simulink model "TRT_sim2021a"  (R2021a)
settings: Solver=VariableStepAuto  StartTime=0.0  StopTime=10.0  RelTol=1e-3
values from neighbouring files (symbols this model uses):
  g = 9.81    [RTR.m]    (also in TRT.m)
  l2 = 0.3    [RTR.m]    (also in TRT.m)
  l3 = 0.2    [RTR.m]    (also in TRT.m)
  m2 = 20    [RTR.m]    (also in TRT.m)
  m3 = 20    [RTR.m]    (also in TRT.m)
settings Model: Creator=kacpe  LastModifiedBy=kacpe
settings DebuggingCC: UnconnectedInputMsg=none  UnconnectedOutputMsg=none  UnconnectedLineMsg=none
settings RTWCC: DLArmComputeVersion=20.02.1

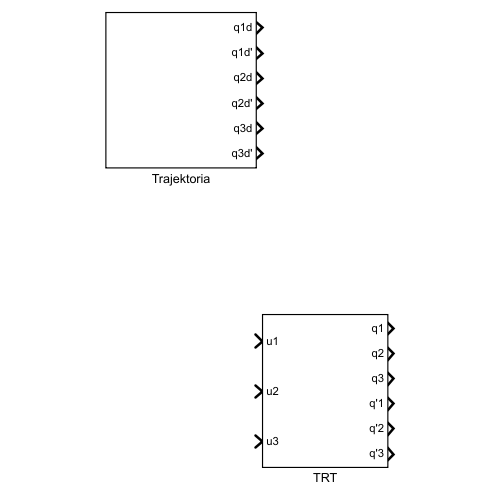
[thumbnail: Simulink's stored preview of the top-level diagram]
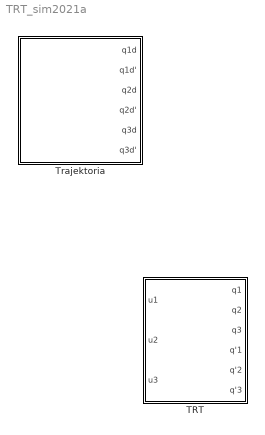
== system TRT_sim2021a ==
  TRT : Subsystem
  Trajektoria : Subsystem

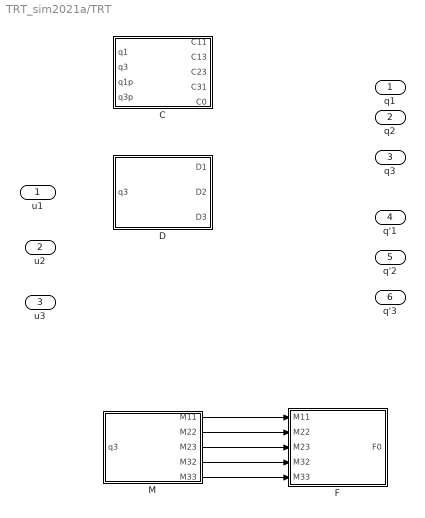
== system TRT_sim2021a/TRT ==
  u1 : Inport
  u2 : Inport  Port=2
  u3 : Inport  Port=3
  C : MATLAB Function  TreatAsAtomicUnit=on
  D : MATLAB Function  TreatAsAtomicUnit=on
  F : MATLAB Function  TreatAsAtomicUnit=on
  M : MATLAB Function  TreatAsAtomicUnit=on
  q1 : Outport
  q2 : Outport  Port=2
  q3 : Outport  Port=3
  q'1 : Outport  Port=4
  q'2 : Outport  Port=5
  q'3 : Outport  Port=6
  wires:
  M/1(M11) -> F/1(M11)
  M/2(M22) -> F/2(M22)
  M/3(M23) -> F/3(M23)
  M/4(M32) -> F/4(M32)
  M/5(M33) -> F/5(M33)

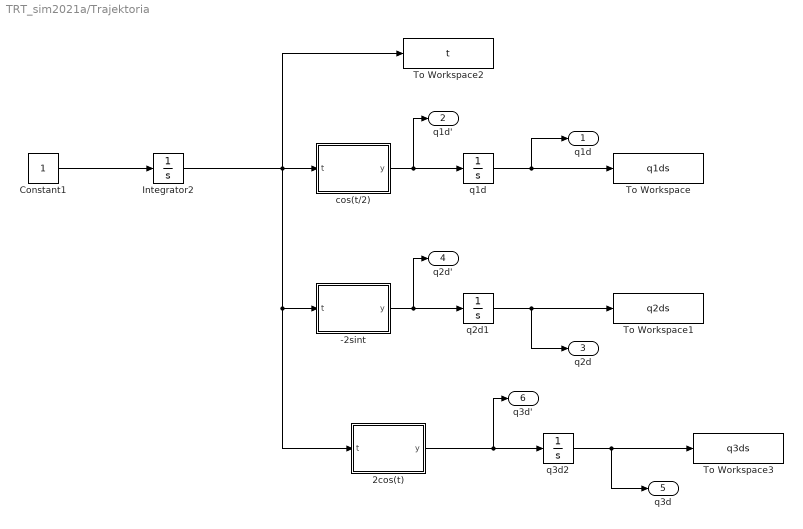
== system TRT_sim2021a/Trajektoria ==
  " q1d" : Integrator
  " q2d1" : Integrator  InitialCondition=2
  " q3d2" : Integrator
  -2sint : MATLAB Function  TreatAsAtomicUnit=on
  2cos(t) : MATLAB Function  TreatAsAtomicUnit=on
  Constant1 : Constant
  Integrator2 : Integrator
  To Workspace : ToWorkspace  VariableName=q1ds  SampleTime=-1
  To Workspace1 : ToWorkspace  VariableName=q2ds  SampleTime=-1
  To Workspace2 : ToWorkspace  VariableName=t  SampleTime=-1
  To Workspace3 : ToWorkspace  VariableName=q3ds  SampleTime=-1
  cos(t/2) : MATLAB Function  TreatAsAtomicUnit=on
  q1d : Outport
  q1d' : Outport  Port=2
  q2d : Outport  Port=3
  q2d' : Outport  Port=4
  q3d : Outport  Port=5
  q3d' : Outport  Port=6
  wires:
  " q2d1"/1 -> To Workspace1/1, q2d/1
  -2sint/1(y) -> q2d'/1, " q2d1"/1
  " q1d"/1 -> To Workspace/1, q1d/1
  cos(t/2)/1(y) -> q1d'/1, " q1d"/1
  Constant1/1 -> Integrator2/1
  Integrator2/1 -> To Workspace2/1, 2cos(t)/1(t), -2sint/1(t), cos(t/2)/1(t)
  " q3d2"/1 -> To Workspace3/1, q3d/1
  2cos(t)/1(y) -> q3d'/1, " q3d2"/1

== matlab function TRT_sim2021a/Trajektoria/2cos(t) ==
  data: t input; y output
function y = fcn(t)

y = 2*cos(t);

== matlab function TRT_sim2021a/TRT/M ==
  data: l2 parameter; l3 parameter; m2 parameter; m3 parameter; q3 input; M11 output; M22 output; M23 output; M32 output; M33 output
function [M11, M22, M23, M32, M33] =fcn(l2,l3, m2, m3, q3)
%(wiersz, kolumna)
%M11, M22,  M33, M23, M32
%% output
%M=[0,0,0;0,0,0;0,0,0];
M11 = (1/3)*m2*(l2^2)+m3*((l2^2)+(1/3)*(l3^2)*(cos(q3)^2) + l2*l3*cos(3));
M22 = m2+m3;
M23 = (1/2)*m3*l2*l3*cos(q3);
M32 = (1/2)*m3*l2*l3*cos(q3);
M33 = (1/3)*m3*(l3^2);
M0=0;

== matlab function TRT_sim2021a/TRT/C ==
  data: q1 input; q3 input; q1p input; q3p input; m3 parameter; l2 parameter; l3 parameter; C11 output; C13 output; C23 output; C31 output; C0 output
function [C11, C13, C23, C31, C0] =fcn( q1, q3, q1p, q3p, m3, l2, l3)
%(wiersz, kolumna)
%M11, M22,  M33, M23, M32
%% output
%M=[0,0,0;0,0,0;0,0,0];
C11 = -q3p*((1/2)*m3*l2*l3*sin(q3) + (1/3)*m3*(l3^2)*sin(q3)*cos*q3);
C13 = -q1p*((1/2)*m3*l2*l3*sin(q3) + (1/3)*m3*(l3^2)*sin(q3)*cos*q3);
C23 = -q3p*(1/2)*m3*(l3^2)*sin(q3)*cos(q3);
C31 = q1p*((1/2)*m3*l2*l3*sin(q3) + (1/3)*m3*(l3^2)*sin(q3)*cos*q3);

== matlab function TRT_sim2021a/TRT/D ==
  data: q3 input; m2 parameter; m3 parameter; l3 parameter; g parameter; D1 output; D2 output; D3 output
function [D1, D2, D3] =fcn(q3,m2,m3, l3, g)
%(wiersz, kolumna)
%M11, M22,  M33, M23, M32
%% output
%M=[0,0,0;0,0,0;0,0,0];
D1 = 0;
D2 = (m2+m3)*g;
D3 = (1/2)*g*m3*l3*cos(q3);

== matlab function TRT_sim2021a/Trajektoria/cos(t//2) ==
  data: t input; y output
function y = fcn(t)

y = cos(t/2);

== matlab function TRT_sim2021a/Trajektoria/-2sint ==
  data: t input; y output
function y = fcn(t)

y = -2*sin(t);

== matlab function TRT_sim2021a/TRT/F ==
  data: M11 input; M22 input; M23 input; F0 output; M32 input; M33 input
function F0  =fcn(M11, M22, M23, M32, M33)
%(wiersz, kolumna)
%M11, M22,  M33, M23, M32
%% output
%M=[0,0,0;0,0,0;0,0,0];
Fpom=inv([1 1 1; 1 1 1; 1 1 1]);


F0 = det(Fpom);
